simulink model "sdrzQPSKTxFPGAretarget"  (R2016a)
settings: Solver=FixedStepDiscrete  SolverMode=SingleTasking  StartTime=0.0  StopTime=inf  RelTol=1e-3
PreLoadFcn:
  | sdrzQPSKTxFPGAretarget_params = sdrzQPSKTxFPGA_init();
InitFcn:
  | sdrzQPSKTxFPGAretarget_params = sdrzQPSKTxFPGA_init();
libraries: dspsigops x2, commrandsrc3 x1, commsequence2 x1, sdrzblksprivate x1, sdrzlib x1
CloseFcn:
  | clear sdrzQPSKTxFPGAretarget_params;
Description:
  | This model uses a targeted .bit generated from the sdrzQPSKTxFPGA example to transmit a QPSK signal using SDR hardware
settings Model: DataTypeOverride=Off  ModifiedByFormat=The MathWorks Inc.  SimulationMode=accelerator  Creator=The MathWorks, Inc.  LastModifiedBy=The MathWorks Inc.
settings DataIOCC: LimitDataPoints=on  SaveFormat=Array  SaveOutput=off  SaveTime=off
settings OptimizationCC: BlockReduction=off  ConditionallyExecuteInputs=off  DefaultParameterBehavior=Inlined
settings DebuggingCC: AlgebraicLoopMsg=error  UnderspecifiedInitializationDetection=Classic  MergeDetectMultiDrivingBlocksExec=none  SolverPrmCheckMsg=warning  MultiTaskDSMMsg=warning  MultiTaskCondExecSysMsg=none  SingleTaskRateTransMsg=error  ParameterPrecisionLossMsg=none  AllowSymbolicDim=off  StateNameClashWarn=warning
settings HardwareCC: ProdBitPerPointer=32  ProdLargestAtomicFloat=None  ProdIntDivRoundTo=Undefined  ProdEndianess=Unspecified  ProdWordSize=32  ProdHWDeviceType=ASIC/FPGA->ASIC/FPGA  ProdEqTarget=off
settings ModelReferenceCC: PropagateSignalLabelsOutOfModel=off
settings ConfigComp: CovModelRefEnable=Off  CovSFcnEnable=off

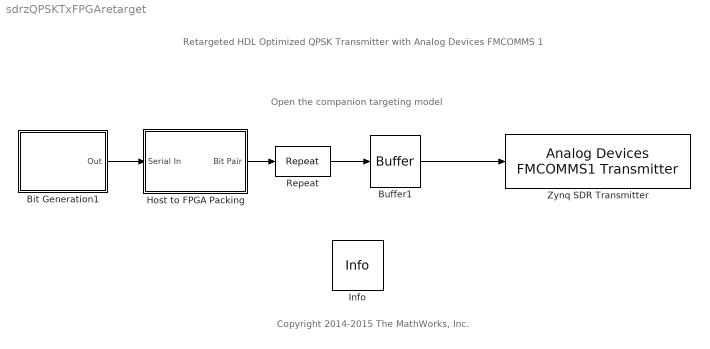
== system sdrzQPSKTxFPGAretarget ==
  note: Copyright 2014-2015 The MathWorks, Inc.
  note: Retargeted HDL Optimized QPSK Transmitter
      | with Analog Devices FMCOMMS 1
  note: Open the companion targeting model
  Bit Generation1 : Subsystem
      mask Display: disp('Bits Generation')
  Buffer1 : Buffer  N=4000  TreatMby1Signals=One channel  OutputFrames=off
  Host to FPGA Packing : Subsystem
  Info : sdrzblksprivate/Info  SystemSampleTime=-1
  Repeat : dspsigops/Repeat  N=sdrzQPSKTxFPGAretarget_params.Upsampling  InputProcessing=Columns as channels (frame based)  RateOptions=Allow multirate processing  ic=0  mode=Unused parameter value
  Zynq SDR Transmitter : sdrzlib/Analog Devices FMCOMMS1 Transmitter  SourceLibraryInfo="This block requires Communications System Toolbox Support Package for Xilinx FPGA-Based Radio. <a href=\"http://www.mathworks.com/hardware-support-packages\">More information</a>"  sobjType=comm.SDRZynqFMCOMMS1Transmitter  IPAddress=192.168.3.2  dataUDPPort=-1  ctrlUDPPort=-1  subDeviceList=comm.SDRZynqFMCOMMS1Transmitter  sdrBlockType=SDRBlockTypeSLT.SDRTxBlock  requester=UNUSED_BY_SFCN  sdrExecutionMode=HW  LostSamplesOutputPort=off  OutputDataType=int16  FrameLength=3660  EnableBurstMode=off  NumFramesInBurst=20  BypassUserLogic=off  InterpolatorSelect=DUC interpolator  SourceSelect=RF data  SineAmplitude=16000  SineFrequency=30000  EnableInternalClock=off  BypassIQBalance=off  CenterFrequencySource=Dialog  CenterFrequency=sdrzQPSKTxFPGAretarget_params.RadioCenterFrequency  IntermediateFrequencySource=Dialog  IntermediateFrequency=sdrzQPSKTxFPGAretarget_params.RadioIntermediateFrequency  IFBandwidthSource=Dialog  IFBandwidth=40e6  DACRateSource=Dialog  DACRate=sdrzQPSKTxFPGAretarget_params.RadioDACRate  GainSource=Dialog  Gain=4.5  InterpolationFactorSource=Dialog  InterpolationFactor=sdrzQPSKTxFPGAretarget_params.RadioInterpolationFactor  RFFrequencyIsTunable=logical(0)  SampleTime=0  BypassDCBlockingFilter=off  IQBalanceCoefficients=64  SkipAllHardwareResetAndInitialization=off  EnableIQCalibrationTable=on  CacheIQCalibrationTable=off
  wires:
  Bit Generation1/1(Out) -> Host to FPGA Packing/1(Serial In)
  Host to FPGA Packing/1(Bit Pair) -> Repeat/1
  Buffer1/1 -> Zynq SDR Transmitter/1
  Repeat/1 -> Buffer1/1

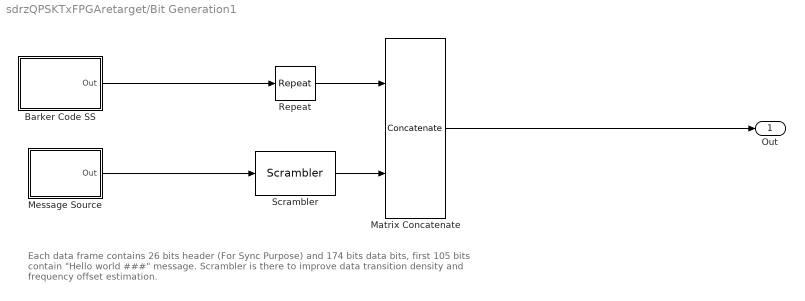
== system sdrzQPSKTxFPGAretarget/Bit Generation1 ==
  note: Each data frame contains 26 bits header (For Sync Purpose) and 174 bits data bits,
      | first 105 bits contain "Hello world ###" message. Scrambler is there to improve data
      | transition density and frequency offset estimation.
  Barker Code SS : Subsystem
      mask Display: disp('Unipolar\nBarker Code')
  Matrix Concatenate : Concatenate  Mode=Multidimensional array
  Message Source : Subsystem
      mask Display: disp('Message\nSource')
  Repeat : dspsigops/Repeat  N=2  InputProcessing=Columns as channels (frame based)  RateOptions=Enforce single-rate processing  ic=0  mode=Unused parameter value
  Scrambler : commsequence2/Scrambler  M=2  poly=[1 1 1 0 1]  iniStaSource=Dialog Parameter  ini_sta=[0 0 0 0]  resetViaPort=off
  Out : Outport
  wires:
  Message Source/1(Out) -> Scrambler/1
  Scrambler/1 -> Matrix Concatenate/2
  Repeat/1 -> Matrix Concatenate/1
  Barker Code SS/1(Out) -> Repeat/1
  Matrix Concatenate/1 -> Out/1

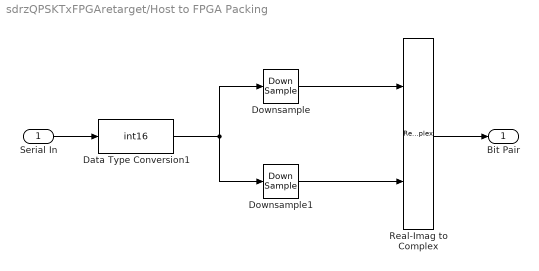
== system sdrzQPSKTxFPGAretarget/Host to FPGA Packing ==
  Serial In : Inport
  Data Type Conversion1 : DataTypeConversion  OutDataTypeStr=int16
  Downsample : DownSample  RateOptions=Allow multirate processing
  Downsample1 : DownSample  phase=1  RateOptions=Allow multirate processing
  Real-Imag to Complex : RealImagToComplex
  Bit Pair : Outport
  wires:
  Real-Imag to Complex/1 -> Bit Pair/1
  Downsample1/1 -> Real-Imag to Complex/2
  Data Type Conversion1/1 -> Downsample/1, Downsample1/1
  Serial In/1 -> Data Type Conversion1/1
  Downsample/1 -> Real-Imag to Complex/1

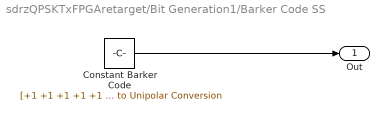
== system sdrzQPSKTxFPGAretarget/Bit Generation1/Barker Code SS ==
  Constant Barker Code : Constant  Value=|  VectorParams1D=off  OutDataTypeStr=double
      | [+1 +1 +1 +1 +1 -1 -1 +1 +1 -1 +1 -1 +1
      | ].' > 0  % Bipolar to Unipolar Conversion
  Out : Outport
  wires:
  Constant Barker Code/1 -> Out/1

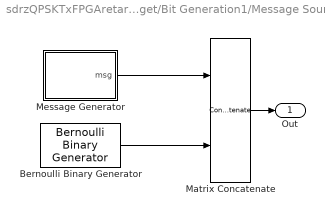
== system sdrzQPSKTxFPGAretarget/Bit Generation1/Message Source ==
  Bernoulli Binary Generator : commrandsrc3/Bernoulli Binary Generator  ProbabilityOfZero=0.5  SeedSource=Parameter  Seed=61  SampleTime=sdrzQPSKTxFPGAretarget_params.FrameTime/(sdrzQPSKTxFPGAretarget_params.DataLength - sdrzQPSKTxFPGAretarget_params.MsgLength)  SamplesPerFrame=sdrzQPSKTxFPGAretarget_params.DataLength - sdrzQPSKTxFPGAretarget_params.MsgLength  OutputDataType=double  SimulateUsing=Interpreted execution
  Matrix Concatenate : Concatenate  Mode=Multidimensional array
  Message Generator : MATLAB Function  TreatAsAtomicUnit=on
  Out : Outport
  wires:
  Matrix Concatenate/1 -> Out/1
  Bernoulli Binary Generator/1 -> Matrix Concatenate/2
  Message Generator/1(msg) -> Matrix Concatenate/1

== matlab function sdrzQPSKTxFPGAretarget/Bit Generation1/Message Source/Message Generator ==
  data: msg output size=[sdrzQPSKTxFPGAretarget_params.MsgLength,1]
function msg = genMsg
%#codegen
persistent msgStrSet count;
if isempty(msgStrSet)
    count = 0;
    msgStrSet = ['Hello world 000';...
              'Hello world 001';...
              'Hello world 002';...
              'Hello world 003';...
              'Hello world 004';...
              'Hello world 005';...
              'Hello world 006';...
              'Hello world 007';...
              'Hello world 008';...
              'Hello world 009';...
              'Hello world 010';...
              'Hello world 011';...
              'Hello world 012';...
              'Hello world 013';...
              'Hello world 014';...
              'Hello world 015';...
              'Hello world 016';...
              'Hello world 017';...
              'Hello world 018';...
              'Hello world 019';...
              'Hello world 020';...
              'Hello world 021';...
              'Hello world 022';...
              'Hello world 023';...
              'Hello world 024';...
              'Hello world 025';...
              'Hello world 026';...
              'Hello world 027';...
              'Hello world 028';...
              'Hello world 029';...
              'Hello world 030';...
              'Hello world 031';...
              'Hello world 032';...
              'Hello world 033';...
              'Hello world 034';...
              'Hello world 035';...
              'Hello world 036';...
              'Hello world 037';...
              'Hello world 038';...
              'Hello world 039';...
              'Hello world 040';...
              'Hello world 041';...
              'Hello world 042';...
              'Hello world 043';...
              'Hello world 044';...
              'Hello world 045';...
              'Hello world 046';...
              'Hello world 047';...
              'Hello world 048';...
              'Hello world 049';...
              'Hello world 050';...
              'Hello world 051';...
              'Hello world 052';...
              'Hello world 053';...
              'Hello world 054';...
              'Hello world 055';...
              'Hello world 056';...
              'Hello world 057';...
              'Hello world 058';...
              'Hello world 059';...
              'Hello world 060';...
              'Hello world 061';...
              'Hello world 062';...
              'Hello world 063';...
              'Hello world 064';...
              'Hello world 065';...
              'Hello world 066';...
              'Hello world 067';...
              'Hello world 068';...
              'Hello world 069';...
              'Hello world 070';...
              'Hello world 071';...
              'Hello world 072';...
              'Hello world 073';...
              'Hello world 074';...
              'Hello world 075';...
              'Hello world 076';...
              'Hello world 077';...
              'Hello world 078';...
              'Hello world 079';...
              'Hello world 080';...
              'Hello world 081';...
              'Hello world 082';...
              'Hello world 083';...
              'Hello world 084';...
              'Hello world 085';...
              'Hello world 086';...
              'Hello world 087';...
              'Hello world 088';...
              'Hello world 089';...
              'Hello world 090';...
              'Hello world 091';...
              'Hello world 092';...
              'Hello world 093';...
              'Hello world 094';...
              'Hello world 095';...
              'Hello world 096';...
              'Hello world 097';...
              'Hello world 098';...
              'Hello world 099'];              
end
msgStr = msgStrSet(count+1,:);
msgBin = de2bi(int8(msgStr),7,'left-msb');
msg = reshape(double(msgBin).',105,1);
count = mod(count+1,100);
